simulink model "ADCS_r2017b"  (R2017b)
settings: Solver=FixedStepAuto  StartTime=0.0  StopTime=end_time  FixedStep=delta_t  RelTol=1e-3
undefined symbols (not defined in the file or in its folder): delta_t, SC, SS
libraries: sharedutil x5, vrlib x2
(part 3 of 3)

== matlab function ADCS_r2017b/Satellite Simulator/External Forces and Torques/External Forces/Moon Gravity ==
  data: r_eci input; a_Moon_eci output; JD input; moon_eci input; GM_moon input
function a_Moon_eci  = moon_gravity(r_eci,JD, moon_eci, GM_moon)

% Reference: Montenbruck (p72)

% T=JD/36525;   
% L_0=218.31617+481267.88088*T-1.3972*T;  %[deg] Moon's mean longitude
% l=134.96272+477198.86753*T;             %[deg] Moon's mean anomaly
% l_prime=357.52543+35999.04944*T;        %[deg] Sun's mean anomaly
% F=93.27283+483202.01873*T;              %[deg] Mean angular distance of Moon from the ascending node
% D=297.85027+445267.11135*T;             %[deg] Difference between the mean longitudes of th Sun and the Moon
% Lambda_M=L_0+22640/60/60*sin(l*pi/180)+769/60/60*sin(2*l*pi/180)...
%          -4586/60/60*sin((l-2*D)*pi/180)+2370/60/60*sin(2*D*pi/180)...
%          -668/60/60*sin((l_prime)*pi/180)-412/60/60*sin(2*F*pi/180)...
%          -212/60/60*sin((2*l-2*D)*pi/180)-206/60/60*sin((l+l_prime-2*D)*pi/180)...
%          +192/60/60*sin((l+2*D)*pi/180)-165/60/60*sin((l_prime-2*D)*pi/180)...
%          +148/60/60*sin((l-l_prime)*pi/180)-125/60/60*sin(D*pi/180)...
%          -110/60/60*sin((l+l_prime)*pi/180)-55/60/60*sin((2*F-2*D)*pi/180); %[deg] lunar longitude
%      
% Beta_M=18520/60/60*sin((F+Lambda_M-L_0+412/60/60*sin(2*F*pi/180)+541/60/60*sin(l_prime*pi/180))*pi/180)...  
%          -526/60/60*sin((F-2*D)*pi/180)+44/60/60*sin((l+F-2*D)*pi/180)...
%          -31/60/60*sin((-l+F-2*D)*pi/180)-25/60/60*sin((-2*l+F)*pi/180)...
%          -23/60/60*sin((l_prime+F-2*D)*pi/180)+21/60/60*sin((-l+F)*pi/180)...
%          +11/60/60*sin((-l_prime+F-2*D)*pi/180); %[deg] lunar latitude
%      
% r_M=(385000-20905*cos(l*pi/180)-3699*cos((2*D-l)*pi/180)...
%     -2956*cos(2*D*pi/180)-570*cos(2*l*pi/180)+246*cos((2*l-2*D)*pi/180)...
%     -205*cos((l_prime-2*D)*pi/180)-171*cos((l+2*D)*pi/180)...
%     -152*cos((l+l_prime-2*D)*pi/180))*1000;  %[m] Distance to Moon
% 
% epsilon=23.43929111; %[deg] equator-ecliptic inclinaison
% 
% Transfomat=[1 0 0;
%             0 cos(epsilon*pi/180) -sin(epsilon*pi/180);
%             0 sin(epsilon*pi/180) cos(epsilon*pi/180)];
% moon_spherical=[r_M*cos(Lambda_M*pi/180)*cos(Beta_M*pi/180);
%             r_M*sin(Lambda_M*pi/180)*cos(Beta_M*pi/180);
%             r_M*sin(Beta_M*pi/180)];
% moon_eci=Transfomat*moon_spherical;

% we calculate moon_eci differently so don't need that code, be consistent

%GM_moon = 4902.801*1E9;		%[m3/s2] Gravity parameter (mu)

mag_dif=((moon_eci(1,1)-r_eci(1,1))^2+(moon_eci(2,1)-r_eci(2,1))^2+(moon_eci(3,1)-r_eci(3,1))^2)^(3/2);
mag=(moon_eci(1,1)^2+moon_eci(2,1)^2+moon_eci(3,1)^2)^(3/2);
a_moon_1=GM_moon*((moon_eci(1,1)-r_eci(1,1))/mag_dif-moon_eci(1,1)/mag);
a_moon_2=GM_moon*((moon_eci(2,1)-r_eci(2,1))/mag_dif-moon_eci(2,1)/mag);
a_moon_3=GM_moon*((moon_eci(3,1)-r_eci(3,1))/mag_dif-moon_eci(3,1)/mag);
a_Moon_eci=[a_moon_1;a_moon_2;a_moon_3];

== matlab function ADCS_r2017b/Satellite Simulator/External Forces and Torques/External Forces/Solar Radiation Pressure ==
  data: r_eci input; a_srp output; sun_eci input; R_eci2body input; eclipse input; unitPtVec input; area_per_face input; mass input; Ca input; Cs input; Cd input
function a_srp = srp(r_eci, sun_eci, R_eci2body, eclipse, unitPtVec, area_per_face,mass, Ca, Cs, Cd)

sat2sun_eci = sun_eci - r_eci;
sat2sun_eci_unit = sat2sun_eci ./ norm(sat2sun_eci);
S = R_eci2body * sat2sun_eci_unit; % unit vector to the sun in body frame

c = 299792458; %m/s
solar_flux = 1361 * (149598023000^2)/(norm(sat2sun_eci)^2); %W/m2
P = solar_flux / c; % solar constant, 

num_faces = length(area_per_face);
a_srp = zeros(3, num_faces);

for i = 1:num_faces
    A = area_per_face(i);
    N = unitPtVec(:,i);
    cos_theta_sun = dot(S, N);
    
    if (cos_theta_sun > 0) && (~eclipse) % surface is illuminated
        a_srp(:,i) = 1/mass*(-P*cos_theta_sun*A * (Ca*S + 2*(Cs*cos_theta_sun + Cd/3)*N));
    end
end
end



% function a_body = srp(r_eci, sun_eci, R_eci2body, eclipse, unitPtVec, area_per_face,mass)
% sat2sun_eci = sun_eci - r_eci;
% sat2sun_eci_unit = sat2sun_eci / norm(sat2sun_eci);
% solar_flux = 1361 * (149598023000^2)/(norm(sat2sun_eci)^2); %W/m2
% sun_dir_body = R_eci2body * sat2sun_eci_unit;
% num_faces = length(area_per_face); %should be 6
% c = 299792458; %m/s
% 
% F = [0;0;0];
% for i=1:num_faces
%     projected_area = area_per_face(i) * dot(unitPtVec(:,i), sun_dir_body);
%     if(projected_area < 0)  %face is not facing sun
%         projected_area = 0;
%     end
%     P = solar_flux/c; %N/m2 
%     F = F+P*projected_area;
% end
% 
% if eclipse
%     a_body = [0;0;0];
% else
%     a_body = (1/mass)*F;
% end

== matlab function ADCS_r2017b/Satellite Simulator/External Forces and Torques/External Forces/Sun Gravity ==
  data: r_eci input; a_Sun_eci output; sun_eci input; GM_sun input
function a_Sun_eci  = sun_gravity(r_eci, sun_eci, GM_sun)

% % Reference: Montenbruck (p70)
% 
% a=149600000000;  % [m]
% e=0.016709;
% i=0;  % [deg]
% Omeg_plus_omeg=282.94; % [deg]
% T=JD/36525;
% M=357.5256+35999.049*T;
% lambda_sun=Omeg_plus_omeg+M+6892/60/60*sin(M*pi/180)+72/60/60*sin(2*M*pi/180)+1.3972*T; %deg
% r_sun=(149.619-2.499*cos(M*pi/180)-0.021*cos(2*M*pi/180))*1E9; %[m]
% epsilon=23.43929111; %[deg]
% Sun_coord=[r_sun*cos(lambda_sun*pi/180);
%            r_sun*sin(lambda_sun*pi/180)*cos(epsilon*pi/180);
%            r_sun*sin(lambda_sun*pi/180)*sin(epsilon*pi/180)];  %ECI cartesian coordinates
       

%GMsun = 1.32712440018e+20;  %[m3/s2] Gravity parameter (mu)  

mag_dif=((sun_eci(1,1)-r_eci(1,1))^2+(sun_eci(2,1)-r_eci(2,1))^2+(sun_eci(3,1)-r_eci(3,1))^2)^(3/2);
mag=(sun_eci(1,1)^2+sun_eci(2,1)^2+sun_eci(3,1)^2)^(3/2);
accSun_1=GM_sun*((sun_eci(1,1)-r_eci(1,1))/mag_dif-sun_eci(1,1)/mag);
accSun_2=GM_sun*((sun_eci(2,1)-r_eci(2,1))/mag_dif-sun_eci(2,1)/mag);
accSun_3=GM_sun*((sun_eci(3,1)-r_eci(3,1))/mag_dif-sun_eci(3,1)/mag);
a_Sun_eci=[accSun_1;accSun_2;accSun_3];
end

== matlab function ADCS_r2017b/Satellite Simulator/External Forces and Torques/External Torques/Aero Torque ==
  data: f_aero_body input; tor output; moment_arms input
function tor = fcn(f_aero_body, moment_arms)
tor = [0;0;0];
for i=length(f_aero_body(1,:))
    tor = tor + Skew(moment_arms(:,i))*f_aero_body(:,i);
end
end

function S = Skew(v)

S =[0 -v(3) v(2)
v(3) 0 -v(1)
-v(2) v(1) 0];
end

== matlab function ADCS_r2017b/Flight Software/Subsystems/RCS Controller/3 Axis Controller/EKF/Calc_Measurement_matrix ==
  data: q_est input; H output; sun_expected input; eclipse input; w_est input; star_limit input
function H = fcn(q_est, sun_expected, eclipse, w_est, star_limit)
%given state estimate, expected sun position (ECI)
%return measurement sensitivity matrix
%measurements are sun body xyz; gyro body xyz
sun_expected = sun_expected / norm(sun_expected);
H = zeros(10,7);
q1 = q_est(1); q2 = q_est(2);
q3 = q_est(3); q4 = q_est(4);

temp = [ q1,  q2,  q3;
        -q2,  q1, -q4;
        -q3,  q4,  q1;
         q4,  q3, -q3;
         q2, -q1,  q4;
         q1,  q2,  q3;
        -q4, -q3,  q2;
        -q3,  q4,  q1;
         q3, -q4, -q1;
         q4,  q3, -q2;
         q1,  q2,  q3;
         q2, -q1,  q4];
temp = 2*temp*sun_expected;
x1 = temp(1); x2 = temp( 2); x3 = temp( 3); x4 = temp( 4);
y1 = temp(5); y2 = temp( 6); y3 = temp( 7); y4 = temp( 8);
z1 = temp(9); z2 = temp(10); z3 = temp(11); z4 = temp(12);
H(1:3, 1:4) = [ x1, x2, x3, x4;
                y1, y2, y3, y4;
                z1, z2, z3, z4];
if(eclipse)
    H(1:3, 1:4) = zeros(3,4);
end
H(4:6, 5:7) = eye(3);

if(norm(w_est) < star_limit)
    H(7:10, 1:4) = eye(4);
end
    
end

== matlab function ADCS_r2017b/Flight Software/Subsystems/RCS Controller/3 Axis Controller/EKF/estimate measurements ==
  data: q_est input; y_hat output; w_est input; sun_eci input; eclipse input; sun_pred output; star_limit input
function [y_hat, sun_pred] = fcn(q_est, w_est, sun_eci, eclipse, star_limit)

gyro_pred = w_est; 
Rot = calc_R(q_est);   
if (eclipse > 0.5)
    sun_pred = [0;0;0];
else
    sun_pred = Rot*sun_eci;   
    sun_pred = sun_pred/norm(sun_pred); %normalize, must be direction
end
if( norm(w_est) > star_limit)
    star_pred = [0;0;0;0];
else
    star_pred = q_est/norm(q_est);
end
y_hat = zeros(10,1);
y_hat(1:3) = sun_pred;
y_hat(4:6) = gyro_pred;
y_hat(7:10) = star_pred;
end

function R_eci2body = calc_R(q)
eta=q(4);
e1=q(1);
e2=q(2);
e3=q(3);

R_eci2body = [e1^2-e2^2-e3^2+eta^2, 2*(e1*e2+eta*e3),        2*(e1*e3-eta*e2);
              2*(e1*e2-eta*e3),     -1*e1^2+e2^2-e3^2+eta^2, 2*(e2*e3+eta*e1);
              2*(e1*e3+eta*e2),     2*(e2*e3-eta*e1),        -1*e1^2-e2^2+e3^2+eta^2];
          
end

== matlab function ADCS_r2017b/Flight Software/Subsystems/RCS Controller/3 Axis Controller/EKF/estimate measurements1 ==
  data: q_est input; y_hat output; w_est input; sun_eci input; eclipse input
function y_hat = fcn(q_est, w_est, sun_eci, eclipse)

gyro_pred = w_est; 
Rot = calc_R(q_est);    
if eclipse
    sun_pred = [0;0;0];
else
    sun_pred = Rot*sun_eci;   
    sun_pred = sun_pred/norm(sun_pred); %normalize, must be direction
end
y_hat = zeros(6,1);
y_hat(1:3) = sun_pred;
y_hat(4:6) = gyro_pred;
end

function R_eci2body = calc_R(q)
eta=q(4);
e1=q(1);
e2=q(2);
e3=q(3);

R_eci2body = [e1^2-e2^2-e3^2+eta^2, 2*(e1*e2+eta*e3),        2*(e1*e3-eta*e2);
              2*(e1*e2-eta*e3),     -1*e1^2+e2^2-e3^2+eta^2, 2*(e2*e3+eta*e1);
              2*(e1*e3+eta*e2),     2*(e2*e3-eta*e1),        -1*e1^2-e2^2+e3^2+eta^2];
          
end

== matlab function ADCS_r2017b/Satellite Simulator/External Forces and Torques/External Torques/SRP Torque ==
  data: f_SRP_body input; tor output; moment_arms input
function tor = fcn(f_SRP_body, moment_arms)
tor = [0;0;0];
for i=length(6)
    tor = tor + Skew(moment_arms(:,i))*f_SRP_body(:,i);
end
end

function S = Skew(v)

S =[0 -v(3) v(2)
v(3) 0 -v(1)
-v(2) v(1) 0];
end

== matlab function ADCS_r2017b/Flight Software/Subsystems/RCS Controller/3 Axis Controller/EKF/estimate measurements2 ==
  data: sun_meas input; y_postfit output; gyr_meas input; y_hat input; eclipse input
function y_postfit = fcn(sun_meas, gyr_meas, y_hat, eclipse)
if eclipse
    y = [0;0;0; gyr_meas];
else
    y = [sun_meas; gyr_meas];
end
y_postfit = y - y_hat;
end

== matlab function ADCS_r2017b/Satellite Simulator/Kinematics/Rotation Kinematics/Euler Equations ==
  data: w input; w_dot output; tor input; I input
function w_dot = fcn(w, tor, I)

w_dot = -I\(Skew(w)*I*w-tor);

% w_dot = zeros(size(w));
% wx = w(1); wy = w(2); wz = w(3);
% Ix = I(1,1); Iy = I(2,2); Iz = I(3,3);
% w_dot(1) = (tor(1) - (Iz-Iy)*wx*wz)/Ix;  %update this to work in body axis
% w_dot(2) = (tor(2) - (Ix-Iz)*wz*wx)/Iy;
% w_dot(3) = (tor(3) - (Iy-Ix)*wx*wy)/Iz;
end


function S = Skew(v)
S = [0 -v(3) v(2)
    v(3) 0 -v(1)
    -v(2) v(1) 0];
end

== matlab function ADCS_r2017b/Satellite Simulator/Sensors/Sun sensor model ==
  data: r_eci input; sun_eci input; sun_meas output; R_eci2body input; noise input; eclipse input; unitPtVec input
function sun_meas = fcn(r_eci, sun_eci, R_eci2body, noise, eclipse, unitPtVec)
sat2sun_eci = sun_eci - r_eci;
sat2sun_eci_unit = sat2sun_eci / norm(sat2sun_eci);
solar_flux = 1361 * (149598023000^2)/(norm(sat2sun_eci)^2); %W/m2
sun_dir_body = R_eci2body * sat2sun_eci_unit;
num_faces = length(unitPtVec); %should be 6

sun_meas = zeros(num_faces, 1);
for i=1:num_faces
    P = solar_flux * dot(unitPtVec(:,i), sun_dir_body);
    if(P < 0 || eclipse) %face is wrong direction
        P = 0;
    end
    %add moon albido
    %%%P = P + fxn(moon_position, orientation)
    P = P/1361;
    sun_meas(i) = P; 
end

sun_meas = sun_meas + noise*randn([6,1]);

== matlab function ADCS_r2017b/Satellite Simulator/Sensors/Star tracker model ==
  data: q_actual input; w_body input; q_meas output; noise input; w_limit input; q_bias input
function q_meas = fcn(q_actual, w_body, noise, w_limit, q_bias)

if norm(w_body) > w_limit
    q_meas = [0;0;0;0];
else
    q_meas = q_actual + noise*randn(4,1);
    q_b = q_bias;
    q_b(1:3) = q_bias(2:4);
    q_b(4)   = q_bias(1); %MATLAB function has scalar first
    q_meas=[q_b(4)   q_b(3)  -q_b(2)  -q_b(1);
           -q_b(3)   q_b(4)   q_b(1)  -q_b(2);
            q_b(2)  -q_b(1)   q_b(4)  -q_b(3);
            q_b(1)   q_b(2)   q_b(3)   q_b(4)]*q_meas; 
    
    q_meas = q_meas/norm(q_meas);
end

== matlab function ADCS_r2017b/Satellite Simulator/Time Model/Date2JD ==
  data: date input; JD output
% function JD = fcn(date)
% %NOTE: this is a little off (about 1.2 days). Compare with own version
% 
% year   = date(1);
% month  = date(2);
% day    = date(3);
% hour   = date(4);
% minute = date(5);
% second = date(6);
% 
% % Calendar Date to Modified Julian Date
% % From Montenbruck, Appendix A, page 321
% 
% % adjust for leap years
% if month <=2
%     y = year - 1;
%     m = month + 12;
% else
%     y = year;
%     m = month;
% end
% 
% % leap days -- ASSUMPTION: we are beyond 4 Oct. 1582
% B = y/400 - y/100 + y/4;
% 
% D = day + hour/24 + minute/(24*60) + second/(24*60*60);
% 
% MJD = 365*y - 679004 + B + (30.6001*(m+1)) + D;
% JD = MJD + 2400000.5;
% end


% %replace this with real function, find text book reference from 279a
% JD_Jan0_2020 = 2458848.5000;
% JD = JD_Jan0_2020 + (year-2020)*365 + month*30 + day + hour/24 + minute/(24*60) + second/(24*60*60);

function JD   = CAL2MJD( date )
%INPUT: Calendar date, MM,DD,YYYY
%OUTPUT: Modified Julian Date, MJD
%source: Montenbruck A.1.1 page 321
Y = date(1);
M = date(2);
D = date(3);
hr  = date(4);
min = date(5);
sec = date(6);

if(Y < 1583)
    disp('Error, year is out of bounds.')
    JD = 0;
else
    if(M <= 2)
        y = Y-1;
        m = M+12;
    else
        y = Y;
        m = M;
    end
    B = floor(y/400)-floor(y/100)+floor(y/4);
    MJD = 365*y-679004+floor(B)+floor(30.6001*(m+1))+D + hr/24 + min/(24*60) + sec/(24*60*60);
    JD = MJD + 2400000.5;
end
end

== matlab function ADCS_r2017b/Satellite Simulator/Sensors/Gyro model ==
  data: w input; meas output; noise input; bias input
function meas = fcn(w, noise, bias)
meas = [0;0;0];
meas = w + bias + noise*randn(3,1);
end

== matlab function ADCS_r2017b/Flight Software/Subsystems/RCS Controller/Spin Stabilized Controller/RCS Command Determination ==
  data: tor input; max_thrust input; norm_dir input; mom_arm input; cmd output; deadband input; est_tor output
function [cmd, est_tor] = fcn(tor, max_thrust, norm_dir, mom_arm, deadband)
%cmd = zeros(12,1);
A = cross(norm_dir,mom_arm);
cmd = (A\tor)/max_thrust;
scale = max(max(cmd),1);
cmd = cmd/scale;
est_tor = zeros(3,1);
for i=1:12
    est_tor = est_tor + max_thrust*cmd(i)*cross(norm_dir(:,i),mom_arm(:,i));
end
    
    
% if(tor(1) > deadband)
%     cmd( 2) = cmd( 2)+0.25*abs(tor(1))/max_tor;
%     cmd( 3) = cmd( 3)+0.25*abs(tor(1))/max_tor;
%     cmd( 5) = cmd( 5)+0.25*abs(tor(1))/max_tor;
%     cmd(12) = cmd(12)+0.25*abs(tor(1))/max_tor;
% elseif(tor(1) < -1*deadband)
%     cmd( 3) = cmd( 3)+0.25*abs(tor(1))/max_tor;
%     cmd( 6) = cmd( 6)+0.25*abs(tor(1))/max_tor;
%     cmd( 8) = cmd( 8)+0.25*abs(tor(1))/max_tor;
%     cmd(11) = cmd(11)+0.25*abs(tor(1))/max_tor;
% end
% 
% if(tor(2) > deadband)
%     cmd( 3) = cmd( 3)+0.25*abs(tor(2))/max_tor;
%     cmd( 9) = cmd( 9)+0.25*abs(tor(2))/max_tor;
%     cmd( 4) = cmd( 4)+0.25*abs(tor(2))/max_tor;
%     cmd(10) = cmd(10)+0.25*abs(tor(2))/max_tor;
% elseif(tor(2) < -1*deadband)
%     cmd( 1) = cmd( 1)+0.25*abs(tor(2))/max_tor;
%     cmd( 7) = cmd( 7)+0.25*abs(tor(2))/max_tor;
%     cmd( 6) = cmd( 6)+0.25*abs(tor(2))/max_tor;
%     cmd(12) = cmd(12)+0.25*abs(tor(2))/max_tor;
% end
%     
% if(tor(3) > deadband)
%     cmd( 1) = cmd( 1)+0.25*abs(tor(3))/max_tor;
%     cmd(10) = cmd(10)+0.25*abs(tor(3))/max_tor;
%     cmd( 5) = cmd( 5)+0.25*abs(tor(3))/max_tor;
%     cmd( 8) = cmd( 8)+0.25*abs(tor(3))/max_tor;
% elseif(tor(3) < -1*deadband)
%     cmd( 4) = cmd( 4)+0.25*abs(tor(3))/max_tor;
%     cmd( 7) = cmd( 7)+0.25*abs(tor(3))/max_tor;
%     cmd( 2) = cmd( 2)+0.25*abs(tor(3))/max_tor;
%     cmd(11) = cmd(11)+0.25*abs(tor(3))/max_tor;
% end

== matlab function ADCS_r2017b/Flight Software/Subsystems/RCS Controller/Spin Stabilized Controller/EKF/Calc_Measurement_matrix ==
  data: q_est input; H output; sun_expected input; eclipse input; w_est input; star_limit input
function H = fcn(q_est, sun_expected, eclipse, w_est, star_limit)
%given state estimate, expected sun position (ECI)
%return measurement sensitivity matrix
%measurements are sun body xyz; gyro body xyz
sun_expected = sun_expected / norm(sun_expected);
H = zeros(10,7);
q1 = q_est(1); q2 = q_est(2);
q3 = q_est(3); q4 = q_est(4);

temp = [ q1,  q2,  q3;
        -q2,  q1, -q4;
        -q3,  q4,  q1;
         q4,  q3, -q3;
         q2, -q1,  q4;
         q1,  q2,  q3;
        -q4, -q3,  q2;
        -q3,  q4,  q1;
         q3, -q4, -q1;
         q4,  q3, -q2;
         q1,  q2,  q3;
         q2, -q1,  q4];
temp = 2*temp*sun_expected;
x1 = temp(1); x2 = temp( 2); x3 = temp( 3); x4 = temp( 4);
y1 = temp(5); y2 = temp( 6); y3 = temp( 7); y4 = temp( 8);
z1 = temp(9); z2 = temp(10); z3 = temp(11); z4 = temp(12);
H(1:3, 1:4) = [ x1, x2, x3, x4;
                y1, y2, y3, y4;
                z1, z2, z3, z4];
if(eclipse)
    H(1:3, 1:4) = zeros(3,4);
end
H(4:6, 5:7) = eye(3);

if(norm(w_est) < star_limit)
    H(7:10, 1:4) = eye(4);
end
    
end


% function H = fcn(q_est, sun_expected, eclipse)
% %given state estimate, expected sun position (ECI)
% %return measurement sensitivity matrix
% %measurements are sun body xyz; gyro body xyz
% sun_expected = sun_expected / norm(sun_expected);
% H = zeros(6,7);
% q1 = q_est(1); q2 = q_est(2);
% q3 = q_est(3); q4 = q_est(4);
% 
% temp = [ q1,  q2,  q3;
%         -q2,  q1, -q4;
%         -q3,  q4,  q1;
%          q4,  q3, -q3;
%          q2, -q1,  q4;
%          q1,  q2,  q3;
%         -q4, -q3,  q2;
%         -q3,  q4,  q1;
%          q3, -q4, -q1;
%          q4,  q3, -q2;
%          q1,  q2,  q3;
%          q2, -q1,  q4];
% temp = 2*temp*sun_expected;
% x1 = temp(1); x2 = temp( 2); x3 = temp( 3); x4 = temp( 4);
% y1 = temp(5); y2 = temp( 6); y3 = temp( 7); y4 = temp( 8);
% z1 = temp(9); z2 = temp(10); z3 = temp(11); z4 = temp(12);
% H(1:3, 1:4) = [ x1, x2, x3, x4;
%                 y1, y2, y3, y4;
%                 z1, z2, z3, z4];
% if(eclipse)
%     H(1:3, 1:4) = zeros(3,4);
% end
% H(4:6, 5:7) = eye(3);
% end

== matlab function ADCS_r2017b/Flight Software/Subsystems/RCS Controller/Spin Stabilized Controller/EKF/estimate measurements ==
  data: q_est input; y_hat output; w_est input; sun_eci input; eclipse input; sun_pred output; star_limit input
function [y_hat, sun_pred] = fcn(q_est, w_est, sun_eci, eclipse, star_limit)

gyro_pred = w_est; 
Rot = calc_R(q_est);   
if (eclipse > 0.5)
    sun_pred = [0;0;0];
else
    sun_pred = Rot*sun_eci;   
    sun_pred = sun_pred/norm(sun_pred); %normalize, must be direction
end
if( norm(w_est) > star_limit)
    star_pred = [0;0;0;0];
else
    star_pred = q_est/norm(q_est);
end
y_hat = zeros(10,1);
y_hat(1:3) = sun_pred;
y_hat(4:6) = gyro_pred;
y_hat(7:10) = star_pred;
end

% function [y_hat, sun_pred] = fcn(q_est, w_est, sun_eci, eclipse)
% 
% gyro_pred = w_est; 
% Rot = calc_R(q_est);   
% if (eclipse > 0.5)
%     sun_pred = [0;0;0];
% else
%     sun_pred = Rot*sun_eci;   
%     sun_pred = sun_pred/norm(sun_pred); %normalize, must be direction
% end
% y_hat = zeros(6,1);
% y_hat(1:3) = sun_pred;
% y_hat(4:6) = gyro_pred;
% end

function R_eci2body = calc_R(q)
eta=q(4);
e1=q(1);
e2=q(2);
e3=q(3);

R_eci2body = [e1^2-e2^2-e3^2+eta^2, 2*(e1*e2+eta*e3),        2*(e1*e3-eta*e2);
              2*(e1*e2-eta*e3),     -1*e1^2+e2^2-e3^2+eta^2, 2*(e2*e3+eta*e1);
              2*(e1*e3+eta*e2),     2*(e2*e3-eta*e1),        -1*e1^2-e2^2+e3^2+eta^2];
          
end

== matlab function ADCS_r2017b/Flight Software/Subsystems/RCS Controller/Spin Stabilized Controller/EKF/estimate measurements1 ==
  data: q_est input; y_hat output; w_est input; sun_eci input; eclipse input
function y_hat = fcn(q_est, w_est, sun_eci, eclipse)

gyro_pred = w_est; 
Rot = calc_R(q_est);    
if eclipse
    sun_pred = [0;0;0];
else
    sun_pred = Rot*sun_eci;   
    sun_pred = sun_pred/norm(sun_pred); %normalize, must be direction
end
y_hat = zeros(6,1);
y_hat(1:3) = sun_pred;
y_hat(4:6) = gyro_pred;
end

function R_eci2body = calc_R(q)
eta=q(4);
e1=q(1);
e2=q(2);
e3=q(3);

R_eci2body = [e1^2-e2^2-e3^2+eta^2, 2*(e1*e2+eta*e3),        2*(e1*e3-eta*e2);
              2*(e1*e2-eta*e3),     -1*e1^2+e2^2-e3^2+eta^2, 2*(e2*e3+eta*e1);
              2*(e1*e3+eta*e2),     2*(e2*e3-eta*e1),        -1*e1^2-e2^2+e3^2+eta^2];
          
end

== matlab function ADCS_r2017b/Flight Software/Subsystems/RCS Controller/Spin Stabilized Controller/EKF/estimate measurements2 ==
  data: sun_meas input; y_postfit output; gyr_meas input; y_hat input; eclipse input
function y_postfit = fcn(sun_meas, gyr_meas, y_hat, eclipse)
if eclipse
    y = [0;0;0; gyr_meas];
else
    y = [sun_meas; gyr_meas];
end
y_postfit = y - y_hat;
end

== matlab function ADCS_r2017b/Flight Software/Subsystems/RCS Controller/Spin Stabilized Controller/EKF/propagate step ==
  data: q_est input; q_out output; w_est input; sigma input; torque input; I input; Q input; w_out output; sigma_out output; dt input
function [q_out, w_out, sigma_out]= fcn(q_est, w_est, sigma, torque, I, Q, dt)
[q_dot, A] = calc_q_dot(q_est, w_est);
w_dot = calc_w_dot(w_est, torque, I);
q = q_est + q_dot * dt;
q_out = q/norm(q);
w_out = w_est + w_dot * dt;
A2 = dt*eye(7); A2(1:4,1:4) = dt*A;
A = calc_A(q_est, w_est, I, dt);
sigma_out = A*sigma*A' + Q;
end

function [q_dot, A] = calc_q_dot(q, w)

wx = w(1); wy = w(2); wz = w(3);
OMEGA = [   0,    wz, -1*wy, wx;
        -1*wz,     0,    wx, wy;
           wy, -1*wx,     0, wz;
        -1*wx, -1*wy, -1*wz,  0];
q_dot = 0.5*OMEGA*q;
A = 0.5*OMEGA; A(1,1)=1; A(2,2)=1; A(3,3)=1; A(4,4)=1;
end

function [w_dot] = calc_w_dot(w, tor, I)

w_dot = -I\(Skew(w)*I*w-tor);

% w_dot = zeros(size(w));
% wx = w(1); wy = w(2); wz = w(3);
% Ix = I(1,1); Iy = I(2,2); Iz = I(3,3);
% w_dot(1) = (tor(1) - (Iz-Iy)*wy*wz)/Ix;  %update this to work in body axis
% w_dot(2) = (tor(2) - (Ix-Iz)*wz*wx)/Iy;
% w_dot(3) = (tor(3) - (Iy-Ix)*wx*wy)/Iz;
end

function S = Skew(v)
S = [0 -v(3) v(2)
    v(3) 0 -v(1)
    -v(2) v(1) 0];
end

function A = calc_A(q, w, I, dt)
wx = w(1); wy = w(2); wz = w(3);
q1 = q(1); q2 = q(2); q3 = q(3); q4 = q(4);
Ix = I(1,1); Iy = I(2,2); Iz = I(3,3);
dti = dt^-1;
A = dt*[  dti,  0.5*wz, -0.5*wy, 0.5*wx,  0.5*q4, -0.5*q3,  0.5*q2;
      -0.5*wz,     dti,  0.5*wx, 0.5*wy,  0.5*q3,  0.5*q4, -0.5*q1; 
       0.5*wy, -0.5*wx,     dti, 0.5*wz, -0.5*q2,  0.5*q1,  0.5*q4;
      -0.5*wx, -0.5*wy, -0.5*wz,    dti, -0.5*q1, -0.5*q2, -0.5*q3;
      0,0,0,0,            dti, -(Iz-Iy)*wz/Ix, -(Iz-Iy)*wy/Ix;
      0,0,0,0, -(Ix-Iz)*wz/Iy,            dti, -(Ix-Iz)*wx/Iy;
      0,0,0,0, -(Iy-Ix)*wy/Iz, -(Iy-Ix)*wx/Iz,            dti]; 

end

== matlab function ADCS_r2017b/Flight Software/Subsystems/RCS Controller/Spin Stabilized Controller/EKF/update_step ==
  data: q_est input; q_out output; w_est input; sigma input; H input; R input; sun_meas input; gyr_meas input; star_meas input; y_hat input; w_out output; sigma_out output; y_prefit output
function [q_out, w_out, sigma_out, y_prefit] = fcn(q_est, w_est, sigma, H, R, sun_meas, gyr_meas, star_meas, y_hat)
y = [sun_meas; gyr_meas; star_meas];
K = sigma*H'*(H*sigma*H'+R)^-1; %Kalman Gain
se = [q_est; w_est];
y_prefit = y - y_hat;
se = se+K*(y_prefit);
sigma_out = (eye(7)-K*H)*sigma*(eye(7)-K*H)'+K*R*K';
q_out = se(1:4);
w_out = se(5:7);
end

== matlab function ADCS_r2017b/Flight Software/Subsystems/RCS Controller/3 Axis Controller/EKF/propagate step ==
  data: q_est input; q_out output; w_est input; sigma input; torque input; I input; Q input; w_out output; sigma_out output; dt input
function [q_out, w_out, sigma_out]= fcn(q_est, w_est, sigma, torque, I, Q, dt)
[q_dot, A] = calc_q_dot(q_est, w_est);
w_dot = calc_w_dot(w_est, torque, I);
q = q_est + q_dot * dt;
q_out = q/norm(q);
w_out = w_est + w_dot * dt;
A2 = dt*eye(7); A2(1:4,1:4) = dt*A;
A = calc_A(q_est, w_est, I, dt);
sigma_out = A*sigma*A' + Q;
end

function [q_dot, A] = calc_q_dot(q, w)

wx = w(1); wy = w(2); wz = w(3);
OMEGA = [   0,    wz, -1*wy, wx;
        -1*wz,     0,    wx, wy;
           wy, -1*wx,     0, wz;
        -1*wx, -1*wy, -1*wz,  0];
q_dot = 0.5*OMEGA*q;
A = 0.5*OMEGA; A(1,1)=1; A(2,2)=1; A(3,3)=1; A(4,4)=1;
end

function [w_dot] = calc_w_dot(w, tor, I)

w_dot = -I\(Skew(w)*I*w-tor);

% w_dot = zeros(size(w));
% wx = w(1); wy = w(2); wz = w(3);
% Ix = I(1,1); Iy = I(2,2); Iz = I(3,3);
% w_dot(1) = (tor(1) - (Iz-Iy)*wy*wz)/Ix;  %update this to work in body axis
% w_dot(2) = (tor(2) - (Ix-Iz)*wz*wx)/Iy;
% w_dot(3) = (tor(3) - (Iy-Ix)*wx*wy)/Iz;
end

function S = Skew(v)
S = [0 -v(3) v(2)
    v(3) 0 -v(1)
    -v(2) v(1) 0];
end

function A = calc_A(q, w, I, dt)
wx = w(1); wy = w(2); wz = w(3);
q1 = q(1); q2 = q(2); q3 = q(3); q4 = q(4);
Ix = I(1,1); Iy = I(2,2); Iz = I(3,3);
dti = dt^-1;
A = dt*[  dti,  0.5*wz, -0.5*wy, 0.5*wx,  0.5*q4, -0.5*q3,  0.5*q2;
      -0.5*wz,     dti,  0.5*wx, 0.5*wy,  0.5*q3,  0.5*q4, -0.5*q1; 
       0.5*wy, -0.5*wx,     dti, 0.5*wz, -0.5*q2,  0.5*q1,  0.5*q4;
      -0.5*wx, -0.5*wy, -0.5*wz,    dti, -0.5*q1, -0.5*q2, -0.5*q3;
      0,0,0,0,            dti, -(Iz-Iy)*wz/Ix, -(Iz-Iy)*wy/Ix;
      0,0,0,0, -(Ix-Iz)*wz/Iy,            dti, -(Ix-Iz)*wx/Iy;
      0,0,0,0, -(Iy-Ix)*wy/Iz, -(Iy-Ix)*wx/Iz,            dti]; 

end

== matlab function ADCS_r2017b/Flight Software/Subsystems/RCS Controller/3 Axis Controller/EKF/update_step ==
  data: q_est input; q_out output; w_est input; sigma input; H input; R input; sun_meas input; gyr_meas input; star_meas input; y_hat input; w_out output; sigma_out output; y_prefit output
function [q_out, w_out, sigma_out, y_prefit] = fcn(q_est, w_est, sigma, H, R, sun_meas, gyr_meas, star_meas, y_hat)
y = [sun_meas; gyr_meas; star_meas];
K = sigma*H'*(H*sigma*H'+R)^-1; %Kalman Gain
se = [q_est; w_est];
y_prefit = y - y_hat;
se = se+K*(y_prefit);
sigma_out = (eye(7)-K*H)*sigma*(eye(7)-K*H)'+K*R*K';
q_out = se(1:4);
w_out = se(5:7);
end

== matlab function ADCS_r2017b/Flight Software/Subsystems/RCS Controller/3 Axis Controller/RCS Command Determination ==
  data: tor input; max_thrust input; norm_dir input; mom_arm input; cmd output; deadband input; est_tor output
function [cmd, est_tor] = fcn(tor, max_thrust, norm_dir, mom_arm, deadband)
%cmd = zeros(12,1);
A = cross(norm_dir,mom_arm);
cmd = (A\tor)/max_thrust;
scale = max(max(cmd),1);
cmd = cmd/scale;
est_tor = [0;0;0];

%apply deadband
%cmd = cmd .* (cmd > deadband);

% for i=1:12
%     est_tor = est_tor + max_thrust*cmd(i)*cross(norm_dir(:,i),mom_arm(:,i));
% end

% if(tor(1) > deadband)
%     cmd( 2) = cmd( 2)+0.25*abs(tor(1))/max_tor;
%     cmd( 3) = cmd( 3)+0.25*abs(tor(1))/max_tor;
%     cmd( 5) = cmd( 5)+0.25*abs(tor(1))/max_tor;
%     cmd(12) = cmd(12)+0.25*abs(tor(1))/max_tor;
% elseif(tor(1) < -1*deadband)
%     cmd( 3) = cmd( 3)+0.25*abs(tor(1))/max_tor;
%     cmd( 6) = cmd( 6)+0.25*abs(tor(1))/max_tor;
%     cmd( 8) = cmd( 8)+0.25*abs(tor(1))/max_tor;
%     cmd(11) = cmd(11)+0.25*abs(tor(1))/max_tor;
% end
% 
% if(tor(2) > deadband)
%     cmd( 3) = cmd( 3)+0.25*abs(tor(2))/max_tor;
%     cmd( 9) = cmd( 9)+0.25*abs(tor(2))/max_tor;
%     cmd( 4) = cmd( 4)+0.25*abs(tor(2))/max_tor;
%     cmd(10) = cmd(10)+0.25*abs(tor(2))/max_tor;
% elseif(tor(2) < -1*deadband)
%     cmd( 1) = cmd( 1)+0.25*abs(tor(2))/max_tor;
%     cmd( 7) = cmd( 7)+0.25*abs(tor(2))/max_tor;
%     cmd( 6) = cmd( 6)+0.25*abs(tor(2))/max_tor;
%     cmd(12) = cmd(12)+0.25*abs(tor(2))/max_tor;
% end
%     
% if(tor(3) > deadband)
%     cmd( 1) = cmd( 1)+0.25*abs(tor(3))/max_tor;
%     cmd(10) = cmd(10)+0.25*abs(tor(3))/max_tor;
%     cmd( 5) = cmd( 5)+0.25*abs(tor(3))/max_tor;
%     cmd( 8) = cmd( 8)+0.25*abs(tor(3))/max_tor;
% elseif(tor(3) < -1*deadband)
%     cmd( 4) = cmd( 4)+0.25*abs(tor(3))/max_tor;
%     cmd( 7) = cmd( 7)+0.25*abs(tor(3))/max_tor;
%     cmd( 2) = cmd( 2)+0.25*abs(tor(3))/max_tor;
%     cmd(11) = cmd(11)+0.25*abs(tor(3))/max_tor;
% end

== matlab function ADCS_r2017b/Flight Software/Subsystems/RCS Controller/Spin Stabilized Controller/Calc_R_eci2mci ==
  data: obliq_e input; R_eci2mci output; obliq_m input
function R_eci2mci = fcn(obliq_e, obliq_m)
ang = (pi/180) * (obliq_e - obliq_m);

%check if this needs to be -1*ang
R_eci2mci = [1,0,0;
             0,cos(ang),-1*sin(ang);
             0,sin(ang),   cos(ang)];
end
